simulink library "motor-propeller dynamics model"  (R2025a)
settings: Solver=VariableStepAuto  StartTime=0.0  StopTime=10.0  RelTol=1e-3
settings Model: Creator=patri  LastModifiedBy=patri

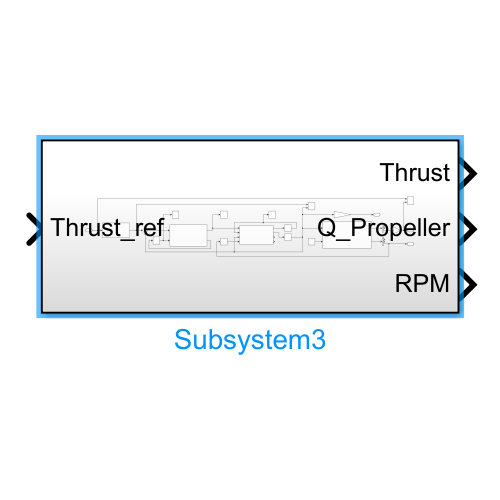
[thumbnail: Simulink's stored preview of the top-level diagram]
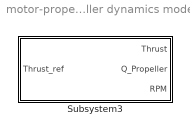
== system motor-propeller dynamics model ==
  Subsystem3 : Subsystem

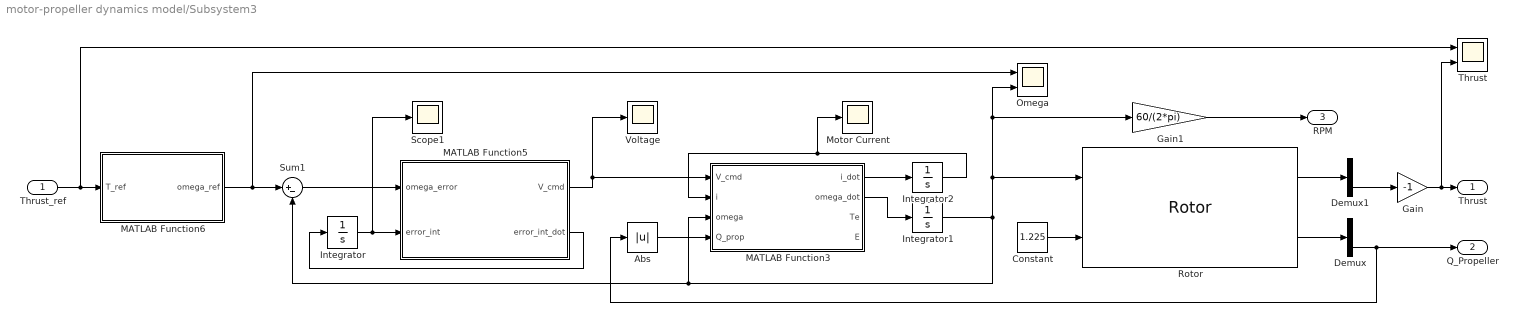
== system motor-propeller dynamics model/Subsystem3 ==
  Thrust_ref : Inport
  Abs : Abs  SaturateOnIntegerOverflow=off
  Constant : Constant  Value=1.225
  Demux : Demux  Outputs=3
  Demux1 : Demux  Outputs=3
  Gain : Gain  Gain=-1
  Gain1 : Gain  Gain=60/(2*pi)
  Integrator : Integrator
  Integrator1 : Integrator
  Integrator2 : Integrator
  MATLAB Function3 : MATLAB Function  TreatAsAtomicUnit=on
  MATLAB Function5 : MATLAB Function  TreatAsAtomicUnit=on
  MATLAB Function6 : MATLAB Function  TreatAsAtomicUnit=on
  Motor Current : Scope
      settings: ActiveDisplayYMinimum=1.7020065933474973  ActiveDisplayYMaximum=6.1259083431162207
  Omega : Scope  NumInputPorts=2
  Rotor : Rotor  CT=0.0165  CQ=0.00214  radius=0.127
  Scope1 : Scope
      settings: ActiveDisplayYMinimum=-1  ActiveDisplayYMaximum=1  DataLoggingVariableName=ScopeData39
  Sum1 : Sum  Inputs=|+-
  "Thrust " : Scope  NumInputPorts=2
      settings: DataLoggingVariableName=ScopeData2
  Voltage : Scope
      settings: ActiveDisplayYMinimum=1.7020065933474973  ActiveDisplayYMaximum=6.1259083431162207  DataLoggingVariableName=ScopeData22
  Thrust : Outport
  Q_Propeller : Outport  Port=2
  RPM : Outport  Port=3
  wires:
  Gain1/1 -> RPM/1
  MATLAB Function3/1(i_dot) -> Integrator2/1
  MATLAB Function5/1(V_cmd) -> Voltage/1, MATLAB Function3/1(V_cmd)
  MATLAB Function6/1(omega_ref) -> Omega/1, Sum1/1
  Sum1/1 -> MATLAB Function5/1(omega_error)
  Thrust_ref/1 -> "Thrust "/1, MATLAB Function6/1(T_ref)
  MATLAB Function5/2(error_int_dot) -> Integrator/1
  Integrator/1 -> Scope1/1, MATLAB Function5/2(error_int)
  MATLAB Function3/2(omega_dot) -> Integrator1/1
  Integrator1/1 -> Omega/2, Gain1/1, Rotor/1, Sum1/2, MATLAB Function3/3(omega)
  Constant/1 -> Rotor/2
  Integrator2/1 -> Motor Current/1, MATLAB Function3/2(i)
  Rotor/2 -> Demux/1
  Abs/1 -> MATLAB Function3/4(Q_prop)
  Demux/3 -> Q_Propeller/1, Abs/1
  Gain/1 -> "Thrust "/2, Thrust/1
  Rotor/1 -> Demux1/1
  Demux1/3 -> Gain/1

== matlab function motor-propeller dynamics model/Subsystem3/MATLAB Function3 ==
  data: V_cmd input; i input; i_dot output; omega input; Q_prop input; omega_dot output; Te output; E output
function [i_dot, omega_dot, Te, E] = motor_dynamics(V_cmd, i, omega, Q_prop)

%% =========================================================
%  DJI 2212 - physical parameters
% ==========================================================

% Nominal voltage
Vnom = 12;                 % [V]

% Electrical parameters
R = 0.25;                  % [ohm]
L = 0.425e-3;              % [H]

% Torque constant
Kt = 18.16e-3;             % [N.m/A]

% Rotor inertia
J = 0.00996e-3;            % [kg.m^2]
% = 9.96e-6 kg.m^2

%% =========================================================
%  Parameters obtained from the no-load operating point
% ==========================================================

I0 = 0.6;                  % no-load current [A]

rpm0 = 10926;              % no-load speed [rpm]

omega0 = rpm0 * 2*pi/60;   % [rad/s]

% Back-EMF
Ke = (Vnom - R*I0)/omega0; % [V.s/rad]

% Equivalent viscous friction
B = Kt*I0/omega0;          % [N.m.s/rad]

%% =========================================================
%  Voltage saturation
% ==========================================================

V = min(max(V_cmd,0),Vnom);

%% =========================================================
%  Electrical dynamics
%
%  V = R*i + L*di/dt + Ke*omega
% ==========================================================

E = Ke*omega;

i_dot = (V - R*i - E)/L;

%% =========================================================
%  Electromagnetic torque
% ==========================================================

Te = Kt*i;

%% =========================================================
%  Mechanical dynamics
%
%  J*domega/dt = Te - B*omega - Q_prop
% ==========================================================

omega_dot = (Te - B*omega - Q_prop)/J;

end

== matlab function motor-propeller dynamics model/Subsystem3/MATLAB Function5 ==
  data: omega_error input; V_cmd output; error_int input; error_int_dot output
function [V_cmd, error_int_dot] = motor_PI_controller(omega_error, error_int)

Kp = 0.02;
Ki = 0.6;

Vmax = 11.1;
Vmin = 0;

% PI control without saturation
V_unsat = Kp*omega_error + Ki*error_int;

% Voltage saturation
V_cmd = min(max(V_unsat, Vmin), Vmax);

% Anti-windup by conditional integration
if (V_unsat >= Vmax && omega_error > 0)
    error_int_dot = 0;

elseif (V_unsat <= Vmin && omega_error < 0)
    error_int_dot = 0;

else
    error_int_dot = omega_error;
end

end

== matlab function motor-propeller dynamics model/Subsystem3/MATLAB Function6 ==
  data: T_ref input; omega_ref output
function omega_ref = thrust_to_omega(T_ref)

rho = 1.225;      % kg/m^3
R   = 0.127;      % 10" / 2 in meters
CT  = 0.0165;

kF = CT*rho*pi*R^4;

T_ref = max(T_ref, 0);

omega_ref = sqrt(T_ref / kF);

end
